simulink model "TpLockInAmp"  (R2020b)
settings: Solver=ode4  StartTime=0.0  StopTime=inf  RelTol=1e-3
undefined symbols (not defined in the file): fdesignblkfcn, gcbh
libraries: dspfdesign x2, dspstat3 x2, dspsrcs4 x2
settings Model: Creator=LYX  LastModifiedBy=LYX
settings OptimizationCC: DefaultParameterBehavior=Inlined  DefaultUnderspecifiedDataType=single  EnhancedBackFolding=on  PassReuseOutputArgsAs=Individual arguments  ZeroExternalMemoryAtStartup=off  ZeroInternalMemoryAtStartup=off  OptimizeBlockOrder=speed  DifferentSizesBufferReuse=on  OptimizationCustomize=off  EfficientTunableParamExpr=on
settings DebuggingCC: ParameterTunabilityLossMsg=error
settings HardwareCC: ProdBitPerPointer=32  ProdBitPerSizeT=32  ProdBitPerPtrDiffT=32  ProdLargestAtomicInteger=Long  ProdWordSize=32  ProdHWDeviceType=ARM Compatible->ARM 7
settings SFSimCC: MATLABDynamicMemAlloc=off
settings RTWCC: Description=Embedded Coder  SystemTargetFile=ert.tlc  GenCodeOnly=on  PackageGeneratedCodeAndArtifacts=on  TemplateMakefile=ert_default_tmf
settings CodeAppCC: ForceParamTrailComments=on  IgnoreCustomStorageClasses=off  OperatorAnnotations=on  SimulinkDataObjDesc=on  SFDataObjDesc=on  InsertBlockDesc=on
settings ERTTargetCC: TargetLangStandard=C99 (ISO)  GenerateSampleERTMain=on  InlinedParameterPlacement=NonHierarchical  ERTCustomFileTemplate=example_file_process.tlc

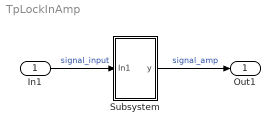
== system TpLockInAmp ==
  In1 : Inport
  Subsystem : Subsystem
  Out1 : Outport
  wires:
  In1/1 -> Subsystem/1(In1)  "signal_input"
  Subsystem/1(y) -> Out1/1  "signal_amp"

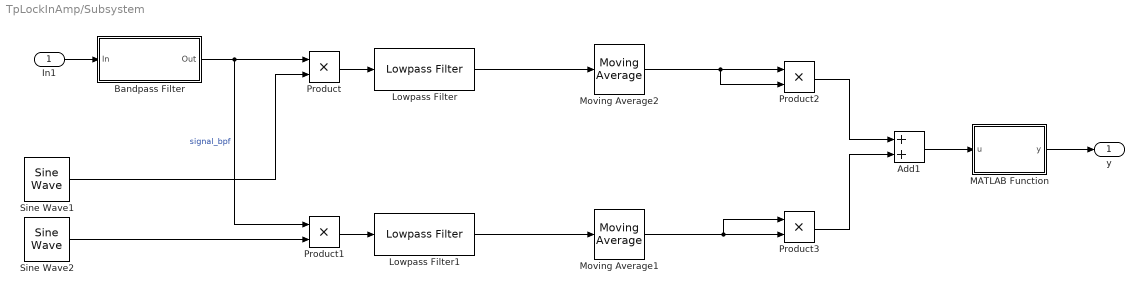
== system TpLockInAmp/Subsystem ==
  In1 : Inport
  Add1 : Sum
  Bandpass Filter : Subsystem  DialogController=fdesignblkfcn  InitFcn=fdesignblkfcn(gcbh, {'InitFcn'});  mask(Bandpass Filter){}
      mask help: Design a bandpass filter
      settings: CopyFcn=fdesignblkfcn(gcbh, {'CopyFcn'});
      mask Help: helpview(mapfilelocation('dsp'), 'dspbandpassfilter');
      mask Display: disp('Bandpass');
  Lowpass Filter : dspfdesign/Lowpass Filter  FilterType=FIR  DesignForMinimumOrder=on  FilterOrder=50  PassbandFrequency=0.3  StopbandFrequency=1.5  PassbandRipple=2  StopbandAttenuation=90  InheritSampleRate=on  SampleRate=240  SimulateUsing=Interpreted execution  roundingMode=Floor  coeffsDataTypeStr=fixdt(1,16)
  Lowpass Filter1 : dspfdesign/Lowpass Filter  FilterType=FIR  DesignForMinimumOrder=on  FilterOrder=50  PassbandFrequency=0.3  StopbandFrequency=1.5  PassbandRipple=2  StopbandAttenuation=90  InheritSampleRate=on  SampleRate=44100  SimulateUsing=Interpreted execution  roundingMode=Floor  coeffsDataTypeStr=fixdt(1,16)
  MATLAB Function : MATLAB Function  TreatAsAtomicUnit=on
  Moving Average1 : dspstat3/Moving Average  Method=Sliding window  ForgettingFactorPort=off  SpecifyWindowLength=on  WindowLength=180  ForgettingFactor=0.9  SimulateUsing=Code generation
  Moving Average2 : dspstat3/Moving Average  Method=Sliding window  ForgettingFactorPort=off  SpecifyWindowLength=on  WindowLength=180  ForgettingFactor=0.9  SimulateUsing=Code generation
  Product{,1..3} (4 alike) : Product
  Sine Wave1 : dspsrcs4/Sine Wave  Amplitude=1  Frequency=20  Phase=0  SampleMode=Discrete  OutComplex=Real  CompMethod=Trigonometric fcn  TableSize=Memory  SampleTime=1/240  SamplesPerFrame=1  ResetState=Restart at time zero  OutputFrames=off  dataType=single  wordLen=16  udDataType=sfix(16)  fracBitsMode=Best precision  numFracBits=15  OutDataTypeStr=single  LastOutDataTypeStr=single
  Sine Wave2 : dspsrcs4/Sine Wave  Amplitude=1  Frequency=20  Phase=pi/2  SampleMode=Discrete  OutComplex=Real  CompMethod=Trigonometric fcn  TableSize=Memory  SampleTime=1/240  SamplesPerFrame=1  ResetState=Restart at time zero  OutputFrames=off  dataType=single  wordLen=16  udDataType=sfix(16)  fracBitsMode=Best precision  numFracBits=15  OutDataTypeStr=single  LastOutDataTypeStr=single
  y : Outport
  wires:
  Sine Wave1/1 -> Product/2
  Add1/1 -> MATLAB Function/1(u)
  Sine Wave2/1 -> Product1/2
  Product3/1 -> Add1/2
  Product2/1 -> Add1/1
  MATLAB Function/1(y) -> y/1
  Product/1 -> Lowpass Filter/1
  Product1/1 -> Lowpass Filter1/1
  Lowpass Filter/1 -> Moving Average2/1
  Moving Average2/1 -> Product2/2, Product2/1
  Lowpass Filter1/1 -> Moving Average1/1
  Moving Average1/1 -> Product3/1, Product3/2
  In1/1 -> Bandpass Filter/1(In)
  Bandpass Filter/1(Out) -> Product1/1, Product/1  "signal_bpf"

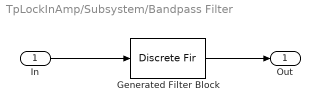
== system TpLockInAmp/Subsystem/Bandpass Filter ==
  In : Inport
  Generated Filter Block : DiscreteFir  Tag=BlockMethodSubSystem  FilterStructure=Direct form symmetric  Coefficients=[9.88985019114446339e-06 -6.85660287976285872e-06 -2.30658676137191028e-05 -3.42685848085714465e-05 -3.70464204728857818e-05 -3.00577501005988695e-05 -1.45511416090330749e-05 5.81218650682615442e-06 2.58204320473895912e-05 4.00565592548811312e-05 4.43770927295934593e-05 3.71173915706188697e-05 1.96721255790565706e-05 -3.74195206516668676e-06 -2.71130142646182268e-05 -4.4199892755225643e-05 -5.02235975569662399e-05 -4.32198315294289928e-05 -2.46651061109857768e-05 8.21351483545599186e-07 2.66457958139584058e-05 4.59794083736962835e-05 5.36023202622261079e-05 4.73446327517703787e-05 2.8717961509123324e-05 2.54900799332331264e-06 -2.42977670873824322e-05 -4.4765335687576202e-05 -5.35110584527228559e-05 -4.8347186603435845e-05 -3.0813918946912344e-05 -5.72609609761376583e-06 2.01766261048486049e-05 4.00933851378946636e-05 4.9012817875594728e-05 4.50313075603467819e-05 2.9775820906975509e-05 7.82910767229842751e-06 -1.46563402790450502e-05 -3.17374520981311803e-05 -3.93281827063288194e-05 -3.62406500450581786e-05 -2.43354236843697027e-05 -7.76983986644919863e-06 8.39405623104257608e-06 1.97714887323420494e-05 2.39293008977601663e-05 2.09640718791508361e-05 1.32260904127984927e-05 4.31085442717703799e-06 -2.32097412279357313e-06 -4.61296049454212541e-06 -2.62735778227771372e-06 1.55190213622070252e-06 4.70510403993497868e-06 3.84871634481396064e-06 -2.39664602316779282e-06 -1.29591539097613301e-05 -2.43551977814956351e-05 -3.16920076159205497e-05 -3.03721682216126515e-05 -1.79623630518811524e-05 4.42806546397227162e-06 3.18176197649163594e-05 5.63363389297860692e-05 6.93721860695778355e-05 6.43203116548402481e-05 3.91056628474156469e-05 -2.37939235696297804e-06 -5.05353432516120939e-05 -9.21578930296245385e-05 -0.000113960643315666661 -0.000106601491371306767 -6.8033828514575662e-05 -5.07803884212943383e-06 6.74702756690610946e-05 0.000130206947308526713 0.000164229794170668304 0.000156666557088897359 0.000105037393417093923 1.90588511590256695e-05 -8.08852218089576577e-05 -0.000168479108655443635 -0.000218347687699589144 -0.000213285442050588369 -0.000149807783214720683 -4.03037572954463534e-05 8.90977168802941722e-05 0.00020468452268554668 0.000273915466128868044 0.000274506220410109967 0.000201325484757537986 6.90203862067679548e-05 -9.06518797247577455e-05 -0.000236394123174283504 -0.000328054573011642137 -0.00033766226598964396 -0.000257783573213200682 -0.000104738259824031145 8.4501134318639215e-05 0.000261219918080527217 0.00037754393012471042 0.000399434216743655899 0.000316558388006935921 0.000146192217831636178 -7.01881906718443069e-05 -0.000277019492839630853 -0.000419003353306992589 -0.000455970067504624327 -0.000374237114573246698 -0.000191248393058038871 4.80069516272071915e-05 0.000282111620784162393 0.000449115338110693942 0.00050306265135583025 0.000426708970604651266 0.000236885502307735004 -1.91302904394375164e-05 -0.00027548721365369932 -0.000464873321897989796 -0.000536379269423656476 -0.000469322735740608618 -0.000279241711995644685 -1.4311903965391757e-05 0.000256998101807736485 0.000463840946856232937 0.000551733591015861032 0.000497108708894690682 0.000313733728315608573 4.92182955565174335e-05 -0.000227505540139578895 -0.000444404033404132944 -0.000545385512510629974 -0.000505058108689880299 -0.000335250203598841281 -8.15761671045838794e-05 0.00018897106211506639 0.000405995223270606516 0.000514350793614269251 0.000488447790278911465 0.00033841628809037406 0.000106602683377652745 -0.000144474436159819131 -0.0003492708108861745 -0.000456699334504137686 -0.000443193315225623636 -0.000317920511110870172 -0.000118968872595770627 9.81470020907548635e-05 0.000276220319039833216 0.000371819231845570315 0.000366209272075104352 0.000268889528600363588 0.000113101956286739249 -5.50134601790246909e-05 -0.00019019196269721365 -0.000260623507514454427 -0.00025575267996703568 -0.000187291042276544915 -8.35554184941568858e-05 2.07410250039986513e-05 9.58212468257987486e-05 0.000125677805472408372 0.00011172364696137728 ...(+14965 chars)]  InputProcessing=Columns as channels (frame based)
  Out : Outport  VectorParamsAs1DForOutWhenUnconnected=off
  wires:
  In/1 -> Generated Filter Block/1
  Generated Filter Block/1 -> Out/1

== matlab function TpLockInAmp/Subsystem/MATLAB Function ==
  data: u input; y output
function y = fcn(u)

y = 2 * sqrt(u);
